simulink model "BPSK"  (R2023a)
settings: Solver=VariableStepAuto  StartTime=0.0  StopTime=10.0  RelTol=1e-3
libraries: commdigbbndpm3 x2, commchan3 x1, commrandsrc3 x1
settings Model: Creator=hh  LastModifiedBy=hh

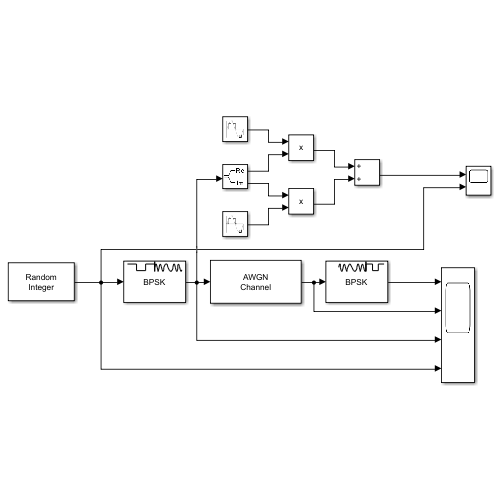
[thumbnail: Simulink's stored preview of the top-level diagram]
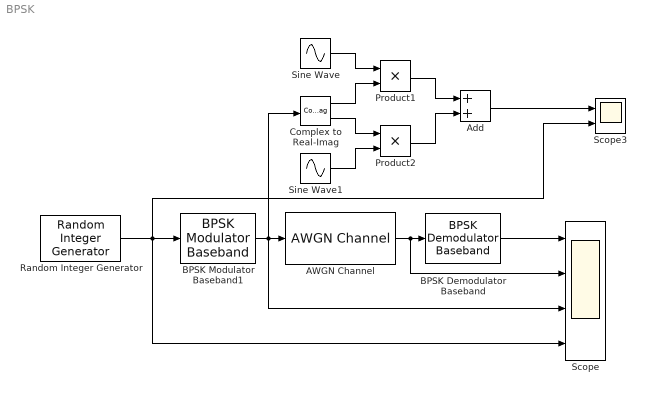
== system BPSK ==
  AWGN Channel : commchan3/AWGN Channel  LegacyMode=off  NoiseMethod="Signal to noise ratio  (SNR)"  noiseMode="Signal to noise ratio  (SNR)"  EbNo=10  EsNo=10  SNR=10  BitsPerSymbol=1  SignalPower=1  SamplesPerSymbol=1  SymbolPeriod=1  VarianceSource=Parameter  Variance=1  RandomStream=Global stream  Seed=67  SimulateUsing=Code generation
  Add : Sum
  BPSK Demodulator Baseband : commdigbbndpm3/BPSK Demodulator Baseband  DecType=Hard decision  VarSource=Dialog  Variance=1  Ph=0  outDtype=Inherit via internal rule  derotateFactorWordLen=16  derotateFactorDataTypeStr=Inherit: Same word length as input  derotateFactorLastDataTypeStr=Inherit: Same word length as input
      settings: LibrarySourceBlock=|
      | commhdldigbbndpm/BPSK
      | Demodulator
      | Baseband
  BPSK Modulator Baseband1 : commdigbbndpm3/BPSK Modulator Baseband  Ph=0  outDtype=double  outWordLen=16  outUDDataType=sfix(16)  outFracLenMode=Best precision  outFracLen=15  outDataTypeStr=double  outLastDataTypeStr=double
  Complex to Real-Imag : ComplexToRealImag
  Product1 : Product
  Product2 : Product
  Random Integer Generator : commrandsrc3/Random Integer Generator  SetSize=2  SeedSource=Auto  Seed=0  SampleTime=1  SamplesPerFrame=1  OutputDataType=uint8  SimulateUsing=Interpreted execution
  Scope : Scope  NumInputPorts=4
  Scope3 : Scope  NumInputPorts=2
  Sine Wave : Sin  Amplitude=4  Frequency=8*pi  SampleTime=0.001
  Sine Wave1 : Sin  Amplitude=4  Frequency=8*pi  Phase=pi/2  SampleTime=0.001
  wires:
  Random Integer Generator/1 -> Scope3/2, Scope/4, BPSK Modulator Baseband1/1
  AWGN Channel/1 -> Scope/2, BPSK Demodulator Baseband/1
  BPSK Demodulator Baseband/1 -> Scope/1
  Product2/1 -> Add/2
  Sine Wave1/1 -> Product2/2
  Product1/1 -> Add/1
  Add/1 -> Scope3/1
  Complex to Real-Imag/2 -> Product2/1
  Sine Wave/1 -> Product1/1
  BPSK Modulator Baseband1/1 -> Complex to Real-Imag/1, Scope/3, AWGN Channel/1
  Complex to Real-Imag/1 -> Product1/2
